simulink model "model4"  (R2019b)
settings: Solver=VariableStepAuto  StartTime=0.0  StopTime=0.3  RelTol=1e-3
libraries: simulink x2
settings Model: Creator=surtweig  LastModifiedBy=surtweig

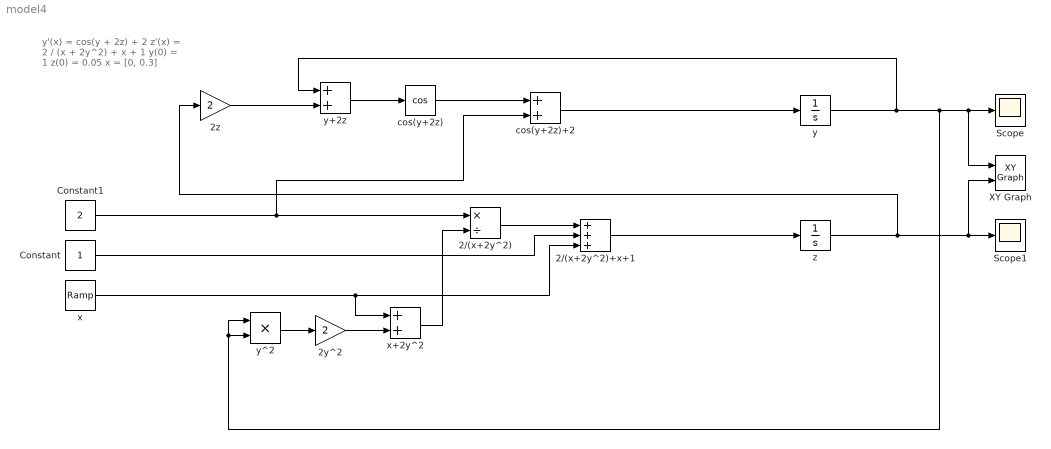
== system model4 ==
  note: y'(x) = cos(y + 2z) + 2
      | z'(x) = 2 / (x + 2y^2) + x + 1
      | y(0) = 1
      | z(0) = 0.05
      | x = [0, 0.3]
  2/(x+2y^2) : Product  Inputs=*/
  2/(x+2y^2)+x+1 : Sum  Inputs=+++
  2y^2 : Gain  Gain=2
  2z : Gain  Gain=2
  Constant : Constant
  Constant1 : Constant  Value=2
  Scope : Scope
  Scope1 : Scope
  XY Graph : simulink/Sinks/XY Graph  xmin=-3  xmax=3  ymin=-3  ymax=3  st=-1
  cos(y+2z) : Trigonometry  Operator=cos
  cos(y+2z)+2 : Sum
  x : simulink/Sources/Ramp  slope=1  start=0  InitialOutput=0
  x+2y^2 : Sum
  y : Integrator  InitialCondition=1
  y+2z : Sum
  y^2 : Product
  z : Integrator  InitialCondition=0.05
  wires:
  y/1 -> y+2z/1, y^2/1, y^2/2, XY Graph/1, Scope/1
  z/1 -> 2z/1, XY Graph/2, Scope1/1
  Constant1/1 -> 2/(x+2y^2)/1, cos(y+2z)+2/2
  x+2y^2/1 -> 2/(x+2y^2)/2
  y^2/1 -> 2y^2/1
  2y^2/1 -> x+2y^2/2
  x/1 -> 2/(x+2y^2)+x+1/3, x+2y^2/1
  2/(x+2y^2)/1 -> 2/(x+2y^2)+x+1/1
  Constant/1 -> 2/(x+2y^2)+x+1/2
  2/(x+2y^2)+x+1/1 -> z/1
  y+2z/1 -> cos(y+2z)/1
  2z/1 -> y+2z/2
  cos(y+2z)/1 -> cos(y+2z)+2/1
  cos(y+2z)+2/1 -> y/1
